simulink library "libraryMatlab"  (R2020b)
settings: Solver=VariableStepAuto  StartTime=0.0  StopTime=10.0  RelTol=1e-3
values from neighbouring files (symbols this model uses):
  data = struct()    [config.m]
undefined symbols (not defined in the file or in its folder): a, SRP
libraries: simulink x2
settings Model: Creator=pacif  LastModifiedBy=pacif

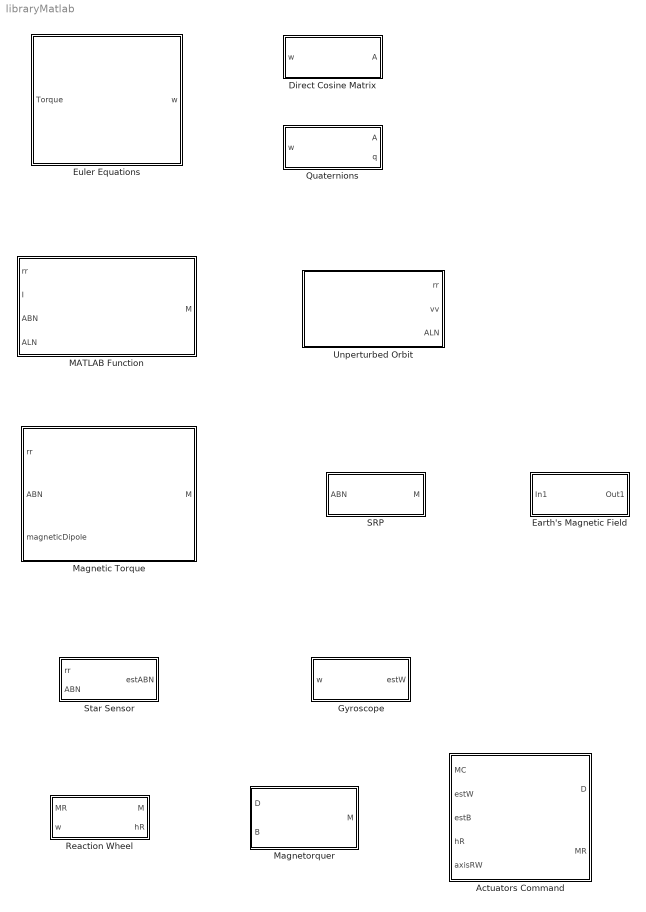
== system libraryMatlab ==
  Actuators Command : MATLAB Function  TreatAsAtomicUnit=on
  Direct Cosine Matrix : Subsystem
  Earth's Magnetic Field : Subsystem
  Euler Equations : Subsystem
  Gyroscope : Subsystem
  MATLAB Function : MATLAB Function  TreatAsAtomicUnit=on
  Magnetic Torque : Subsystem
  Magnetorquer : MATLAB Function  TreatAsAtomicUnit=on
  Quaternions : Subsystem
  Reaction Wheel : Subsystem
  SRP : Subsystem  AncestorBlock=a/SRP
  Star Sensor : Subsystem
  Unperturbed Orbit : Subsystem

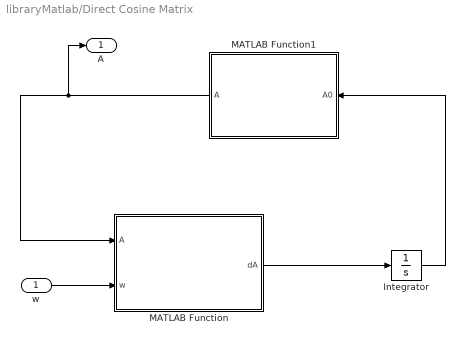
== system libraryMatlab/Direct Cosine Matrix ==
  w : Inport
  Integrator : Integrator  InitialCondition=data.ic.dcm
  MATLAB Function : MATLAB Function  TreatAsAtomicUnit=on
  MATLAB Function1 : MATLAB Function  TreatAsAtomicUnit=on
  A : Outport
  wires:
  w/1 -> MATLAB Function/2(w)
  MATLAB Function/1(dA) -> Integrator/1
  Integrator/1 -> MATLAB Function1/1(A0)
  MATLAB Function1/1(A) -> A/1, MATLAB Function/1(A)

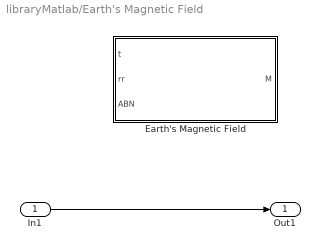
== system libraryMatlab/Earth's Magnetic Field ==
  In1 : Inport
  Earth's Magnetic Field : MATLAB Function  TreatAsAtomicUnit=on
  Out1 : Outport
  wires:
  In1/1 -> Out1/1

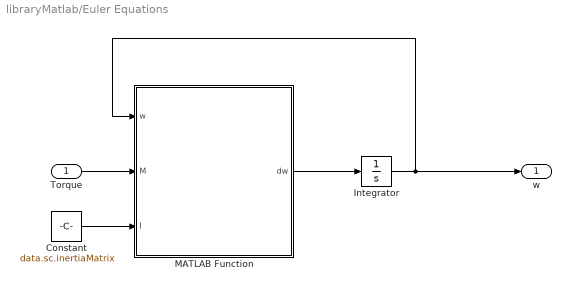
== system libraryMatlab/Euler Equations ==
  Torque : Inport
  Constant : Constant  Value=data.sc.inertiaMatrix
  Integrator : Integrator  InitialCondition=data.ic.w
  MATLAB Function : MATLAB Function  TreatAsAtomicUnit=on
  w : Outport
  wires:
  Constant/1 -> MATLAB Function/3(I)
  Integrator/1 -> w/1, MATLAB Function/1(w)
  Torque/1 -> MATLAB Function/2(M)
  MATLAB Function/1(dw) -> Integrator/1

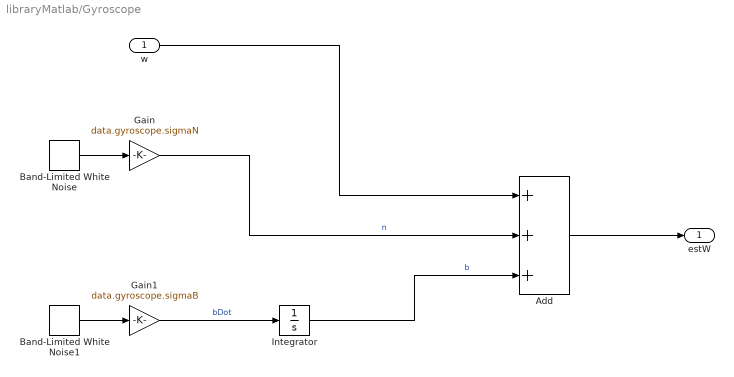
== system libraryMatlab/Gyroscope ==
  w : Inport
  Add : Sum  Inputs=+++
  Band-Limited White Noise : simulink/Sources/Band-Limited White Noise  Cov=[1; 1; 1]  Ts=data.gyroscope.sampleTime  seed=[23341]
  Band-Limited White Noise1 : simulink/Sources/Band-Limited White Noise  Cov=[1; 1; 1]  Ts=data.gyroscope.sampleTime  seed=[23341]
  Gain : Gain  Gain=data.gyroscope.sigmaN
  Gain1 : Gain  Gain=data.gyroscope.sigmaB
  Integrator : Integrator  InitialCondition=[0;0;0]
  estW : Outport
  wires:
  Band-Limited White Noise/1 -> Gain/1
  Gain/1 -> Add/2  "n"
  Gain1/1 -> Integrator/1  "bDot"
  Integrator/1 -> Add/3  "b"
  w/1 -> Add/1
  Add/1 -> estW/1
  Band-Limited White Noise1/1 -> Gain1/1

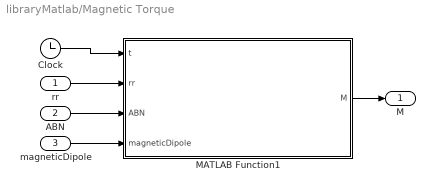
== system libraryMatlab/Magnetic Torque ==
  rr : Inport
  ABN : Inport  Port=2
  magneticDipole : Inport  Port=3
  Clock : Clock
  MATLAB Function1 : MATLAB Function  TreatAsAtomicUnit=on
  M : Outport
  wires:
  MATLAB Function1/1(M) -> M/1
  rr/1 -> MATLAB Function1/2(rr)
  ABN/1 -> MATLAB Function1/3(ABN)
  magneticDipole/1 -> MATLAB Function1/4(magneticDipole)
  Clock/1 -> MATLAB Function1/1(t)

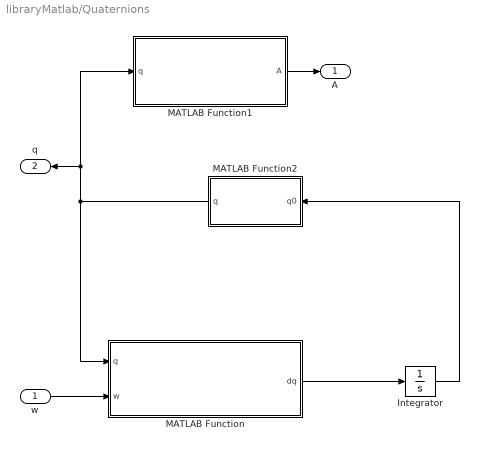
== system libraryMatlab/Quaternions ==
  w : Inport
  Integrator : Integrator  InitialCondition=data.ic.quaternions
  MATLAB Function : MATLAB Function  TreatAsAtomicUnit=on
  MATLAB Function1 : MATLAB Function  TreatAsAtomicUnit=on
  MATLAB Function2 : MATLAB Function  TreatAsAtomicUnit=on
  A : Outport
  q : Outport  Port=2
  wires:
  w/1 -> MATLAB Function/2(w)
  MATLAB Function/1(dq) -> Integrator/1
  Integrator/1 -> MATLAB Function2/1(q0)
  MATLAB Function2/1(q) -> MATLAB Function/1(q), q/1, MATLAB Function1/1(q)
  MATLAB Function1/1(A) -> A/1

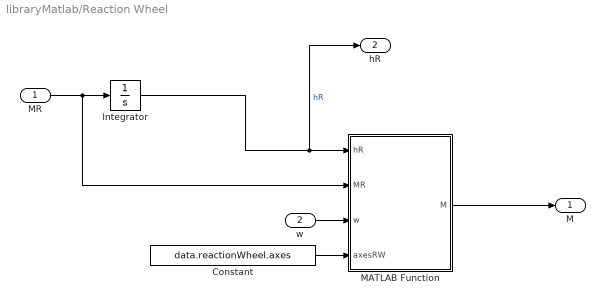
== system libraryMatlab/Reaction Wheel ==
  MR : Inport
  w : Inport  Port=2
  Constant : Constant  Value=data.reactionWheel.axes
  Integrator : Integrator
  MATLAB Function : MATLAB Function  TreatAsAtomicUnit=on
  M : Outport
  hR : Outport  Port=2
  wires:
  MR/1 -> MATLAB Function/2(MR), Integrator/1
  Integrator/1 -> hR/1, MATLAB Function/1(hR)  "hR"
  Constant/1 -> MATLAB Function/4(axesRW)
  w/1 -> MATLAB Function/3(w)
  MATLAB Function/1(M) -> M/1

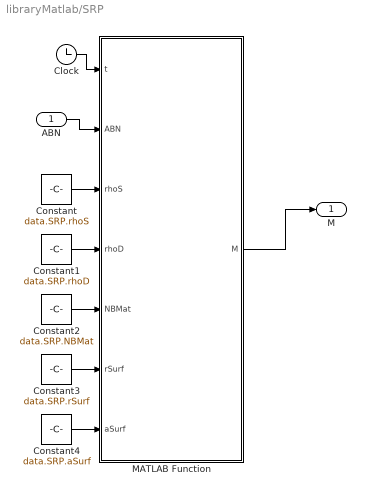
== system libraryMatlab/SRP ==
  ABN : Inport
  Clock : Clock
  Constant : Constant  Value=data.SRP.rhoS
  Constant1 : Constant  Value=data.SRP.rhoD
  Constant2 : Constant  Value=data.SRP.NBMat
  Constant3 : Constant  Value=data.SRP.rSurf
  Constant4 : Constant  Value=data.SRP.aSurf
  MATLAB Function : MATLAB Function  TreatAsAtomicUnit=on
  M : Outport
  wires:
  Constant4/1 -> MATLAB Function/7(aSurf)
  Constant3/1 -> MATLAB Function/6(rSurf)
  Constant2/1 -> MATLAB Function/5(NBMat)
  Constant1/1 -> MATLAB Function/4(rhoD)
  Constant/1 -> MATLAB Function/3(rhoS)
  Clock/1 -> MATLAB Function/1(t)
  MATLAB Function/1(M) -> M/1
  ABN/1 -> MATLAB Function/2(ABN)

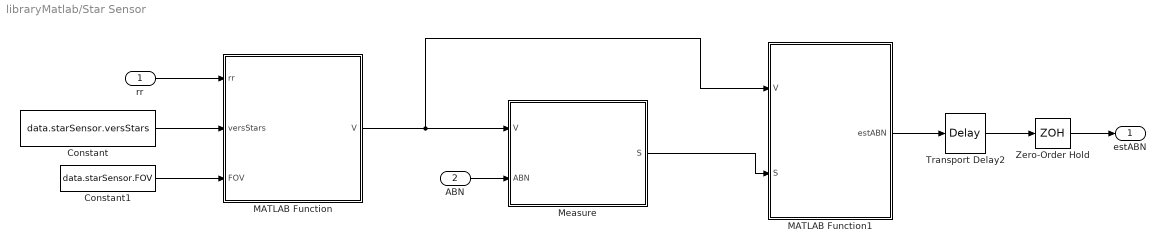
== system libraryMatlab/Star Sensor ==
  rr : Inport
  ABN : Inport  Port=2
  Constant : Constant  Value=data.starSensor.versStars
  Constant1 : Constant  Value=data.starSensor.FOV
  MATLAB Function : MATLAB Function  TreatAsAtomicUnit=on
  MATLAB Function1 : MATLAB Function  TreatAsAtomicUnit=on
  Measure : Subsystem
  Transport Delay2 : TransportDelay  DelayTime=data.starSensor.sampleTime
  Zero-Order Hold : ZeroOrderHold  SampleTime=data.starSensor.sampleTime
  estABN : Outport
  wires:
  Constant/1 -> MATLAB Function/2(versStars)
  Constant1/1 -> MATLAB Function/3(FOV)
  Measure/1(S) -> MATLAB Function1/2(S)
  ABN/1 -> Measure/2(ABN)
  Zero-Order Hold/1 -> estABN/1
  rr/1 -> MATLAB Function/1(rr)
  MATLAB Function/1(V) -> MATLAB Function1/1(V), Measure/1(V)
  MATLAB Function1/1(estABN) -> Transport Delay2/1
  Transport Delay2/1 -> Zero-Order Hold/1

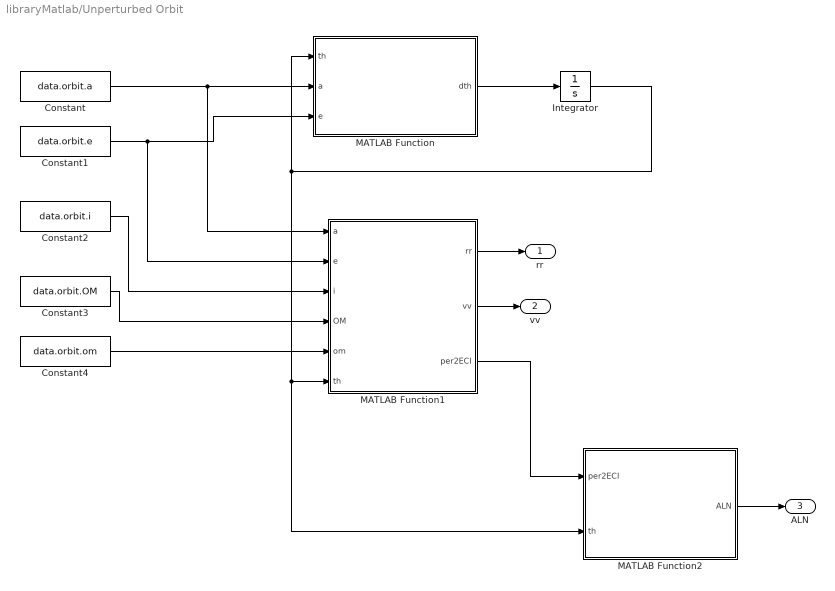
== system libraryMatlab/Unperturbed Orbit ==
  Constant : Constant  Value=data.orbit.a
  Constant1 : Constant  Value=data.orbit.e
  Constant2 : Constant  Value=data.orbit.i
  Constant3 : Constant  Value=data.orbit.OM
  Constant4 : Constant  Value=data.orbit.om
  Integrator : Integrator  InitialCondition=data.ic.th
  MATLAB Function : MATLAB Function  TreatAsAtomicUnit=on
  MATLAB Function1 : MATLAB Function  TreatAsAtomicUnit=on
  MATLAB Function2 : MATLAB Function  TreatAsAtomicUnit=on
  rr : Outport
  vv : Outport  Port=2
  ALN : Outport  Port=3
  wires:
  Constant/1 -> MATLAB Function1/1(a), MATLAB Function/2(a)
  Constant1/1 -> MATLAB Function1/2(e), MATLAB Function/3(e)
  MATLAB Function/1(dth) -> Integrator/1
  Integrator/1 -> MATLAB Function2/2(th), MATLAB Function1/6(th), MATLAB Function/1(th)
  Constant2/1 -> MATLAB Function1/3(i)
  Constant3/1 -> MATLAB Function1/4(OM)
  Constant4/1 -> MATLAB Function1/5(om)
  MATLAB Function1/1(rr) -> rr/1
  MATLAB Function1/2(vv) -> vv/1
  MATLAB Function1/3(per2ECI) -> MATLAB Function2/1(per2ECI)
  MATLAB Function2/1(ALN) -> ALN/1

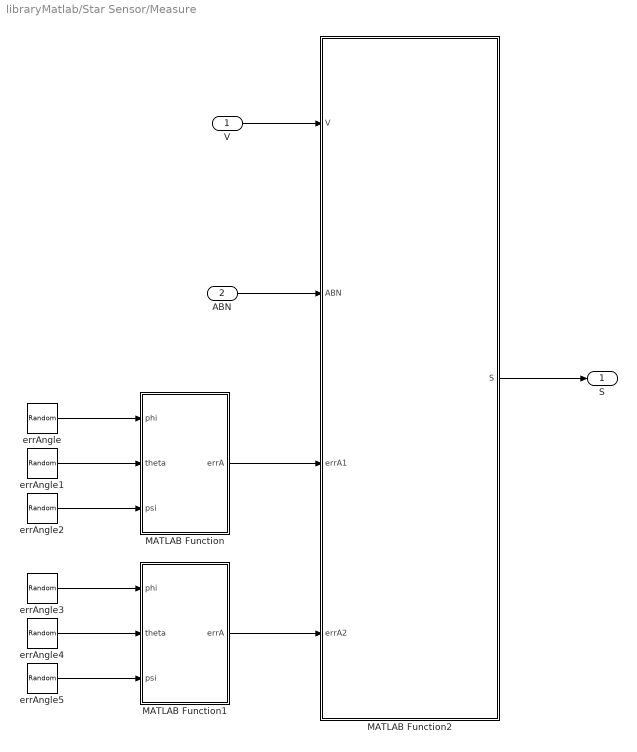
== system libraryMatlab/Star Sensor/Measure ==
  V : Inport
  ABN : Inport  Port=2
  MATLAB Function : MATLAB Function  TreatAsAtomicUnit=on
  MATLAB Function1 : MATLAB Function  TreatAsAtomicUnit=on
  MATLAB Function2 : MATLAB Function  TreatAsAtomicUnit=on
  errAngle{,1..5} (6 alike) : RandomNumber  Variance=data.starSensor.variance  SampleTime=data.starSensor.sampleTime
  S : Outport
  wires:
  errAngle/1 -> MATLAB Function/1(phi)
  errAngle1/1 -> MATLAB Function/2(theta)
  errAngle2/1 -> MATLAB Function/3(psi)
  errAngle5/1 -> MATLAB Function1/3(psi)
  errAngle4/1 -> MATLAB Function1/2(theta)
  errAngle3/1 -> MATLAB Function1/1(phi)
  MATLAB Function/1(errA) -> MATLAB Function2/3(errA1)
  MATLAB Function1/1(errA) -> MATLAB Function2/4(errA2)
  MATLAB Function2/1(S) -> S/1
  V/1 -> MATLAB Function2/1(V)
  ABN/1 -> MATLAB Function2/2(ABN)

== matlab function libraryMatlab/Magnetic Torque/MATLAB Function1 ==
  data: t input; M output; rr input; ABN input; magneticDipole input
function M = magneticTorque(t,rr,ABN,magneticDipole)

% Coefficients for 2020:
g10 = -29615e-9; g11 = -1728e-9; h11 = 5186e-9;
H0 = sqrt(g10^2 + g11^2 + h11^2);

OBL = 11.5*pi/180;
W_EARTH = (2*pi + 2*pi/365.26)/24/3600;
R_EARTH = 6371.0088;

mVers = [sin(OBL)*cos(W_EARTH*t);
        sin(OBL)*sin(W_EARTH*t);
        cos(OBL)];

rVers = rr/norm(rr);
rNorm = norm(rr);

bN = R_EARTH^3/rNorm^3*H0*(3*dot(mVers,rVers)*rVers - mVers);

bB = ABN*bN;

M = cross(magneticDipole,bB); 

end

== matlab function libraryMatlab/SRP/MATLAB Function ==
  data: t input; ABN input; M output; rhoS input; rhoD input; NBMat input; rSurf input; aSurf input
function M = SRP(t,ABN,rhoS,rhoD,NBMat,rSurf,aSurf)

% Constants:
Fe = 2081.4; c = 3e8; P = Fe/c;

N_SUN = 2*pi/365/24/3600; OBL = 23.45*pi/180;
R_SUN = 1.496e8;

SN = R_SUN*[cos(N_SUN*t); 
    sin(N_SUN*t)*cos(OBL);
    sin(N_SUN*t)*sin(OBL)];
SN = SN/norm(SN);

SB = ABN*SN;

nSurf = size(NBMat,2);

M = [0; 0; 0];

for i = 1:nSurf
    
    NBi = NBMat(:,i); ri = rSurf(:,i); Ai = aSurf(i);
    rhoSi = rhoS(i); rhoDi = rhoD(i);
    
    Ki = dot(SB,NBi); 
    
    if Ki > 0
        
        Fi = -P*Ai*Ki*((1-rhoSi)*SB +...
            (2*rhoSi*Ki + 2/3*rhoDi)*NBi);
        
        M = M + cross(ri,Fi);
        
    end
    
end

end

== matlab function libraryMatlab/Star Sensor/MATLAB Function ==
  data: rr input; V output; versStars input; FOV input
function V = starCatalog(rr,versStars,FOV)

rrVers = rr/norm(rr);

% Search on star catalogue:

angles = acos(versStars*rrVers);

anglesInFOV = angles < FOV;

starsInFOV = versStars(anglesInFOV,:);

nMeasures = 2;

V = starsInFOV(1:nMeasures,:)';

== matlab function libraryMatlab/Star Sensor/MATLAB Function1 ==
  data: V input; estABN output; S input
function estABN = attitudeEstimation(V,S)

p = S(:,1); q = S(:,2); a = V(:,1); b = V(:,2);

m1 = p; 
m2 = cross(p,q); m2 = m2/norm(m2);
m3 = cross(p,m2);

n1 = a; 
n2 = cross(a,b); n2 = n2/norm(n2);
n3 = cross(a,n2);

M = [m1, m2, m3]; N = [n1, n2, n3];

estABN = M*N';

== matlab function libraryMatlab/Direct Cosine Matrix/MATLAB Function ==
  data: A input; dA output; w input
function dA = derivativeDCM(A,w)

M = [ 0 -w(3) w(2); 
    w(3) 0 -w(1);
    -w(2) w(1) 0];

dA = -M*A;


end

== matlab function libraryMatlab/Star Sensor/Measure/MATLAB Function ==
  data: phi input; errA output; theta input; psi input
function errA = errorRotation(phi,theta,psi)

errA = [ cos(psi)*cos(theta), cos(phi)*sin(psi) + cos(psi)*sin(phi)*sin(theta), sin(phi)*sin(psi) - cos(phi)*cos(psi)*sin(theta)
-cos(theta)*sin(psi), cos(phi)*cos(psi) - sin(phi)*sin(psi)*sin(theta), cos(psi)*sin(phi) + cos(phi)*sin(psi)*sin(theta)
          sin(theta),                             -cos(theta)*sin(phi),                              cos(phi)*cos(theta)];

== matlab function libraryMatlab/Star Sensor/Measure/MATLAB Function1 ==
  data: phi input; errA output; theta input; psi input
function errA = errorRotation(phi,theta,psi)

errA = [ cos(psi)*cos(theta), cos(phi)*sin(psi) + cos(psi)*sin(phi)*sin(theta), sin(phi)*sin(psi) - cos(phi)*cos(psi)*sin(theta)
-cos(theta)*sin(psi), cos(phi)*cos(psi) - sin(phi)*sin(psi)*sin(theta), cos(psi)*sin(phi) + cos(phi)*sin(psi)*sin(theta)
          sin(theta),                             -cos(theta)*sin(phi),                              cos(phi)*cos(theta)];

== matlab function libraryMatlab/Star Sensor/Measure/MATLAB Function2 ==
  data: V input; S output; ABN input; errA1 input; errA2 input
function S = measure(V,ABN,errA1,errA2)

r1 = V(:,1); r2 = V(:,2);

s1 = errA1*ABN*r1; s2 = errA2*ABN*r2;

S = [s1, s2];

== matlab function libraryMatlab/Reaction Wheel/MATLAB Function ==
  data: hR input; M output; MR input; w input; axesRW input
function M = reactionWheel(hR,MR,w,axesRW)

M = -cross(w,axesRW*hR) - A*MR;

end

== matlab function libraryMatlab/Magnetorquer ==
  data: D input; M output; B input
function M = magnetorquer(D,B)

M = cross(D,B);

end

== matlab function libraryMatlab/Actuators Command ==
  data: MC input; D output; estW input; estB input; hR input; axisRW input; MR output
function [D,MR] = actuatorsCommand(MC, estW, estB, hR, axisRW)

M = MC + cross(estW,hR*axisRW);

Bx = estB(1); By = estB(2); Bz = estB(3);
ax = axisRW(1); ay = axisRW(2); az = axisRW(3);

C = [0, Bz, -By, -ax
     -Bz, 0, Bx, -ay
     By, -Bx, 0, -az];
 
invC = C'*inv(C*C');

u = invC*M;

D = u(1:3); MR = u(4);

end

== matlab function libraryMatlab/Earth's Magnetic Field/Earth's Magnetic Field ==
  data: t input; M output; rr input; ABN input
function M = fcn(t,rr,ABN)

% Coefficients for 2020:
g10 = -29615e-9; g11 = -1728e-9; h11 = 5186e-9;
H0 = sqrt(g10^2 + g11^2 + h11^2);

OBL = 11.5*pi/180;
W_EARTH = (2*pi + 2*pi/365.26)/24/3600;
R_EARTH = 6371.0088;

mVers = [sin(OBL)*cos(W_EARTH*t);
        sin(OBL)*sin(W_EARTH*t);
        cos(OBL)];

rVers = rr/norm(rr);
rNorm = norm(rr);

bN = R_EARTH^3/rNorm^3*H0*(3*dot(mVers,rVers)*rVers - mVers);

bB = ABN*bN;

end

== matlab function libraryMatlab/Euler Equations/MATLAB Function ==
  data: w input; dw output; M input; I input
function dw = eulerEquations(w,M,I)

dw = I\(cross(I*w,w) + M);

end

== matlab function libraryMatlab/Direct Cosine Matrix/MATLAB Function1 ==
  data: A0 input; A output
function A = orthonormalizeA(A0)

A = A0*3/2 - A0*(A0')*A0/2;

end

== matlab function libraryMatlab/Quaternions/MATLAB Function ==
  data: q input; dq output; w input
function dq = derivativeQuaternions(q,w)

w1 = w(1); w2 = w(2); w3 = w(3);

M = [0 w3 -w2 w1; 
    -w3 0 w1 w2;
    w2 -w1 0 w3;
    -w1 -w2 -w3 0];

dq = 0.5*M*q;

end

== matlab function libraryMatlab/Quaternions/MATLAB Function1 ==
  data: q input; A output
function A = quatToDCM(q)

q1 = q(1); q2 = q(2); q3 = q(3); q4 = q(4);

A = [ q1^2-q2^2-q3^2+q4^2    2*(q1*q2+q3*q4)        2*(q1*q3-q2*q4);
    2*(q1*q2-q3*q4)          -q1^2+q2^2-q3^2+q4^2   2*(q2*q3+q1*q4);
    2*(q1*q3+q2*q4)          2*(q2*q3-q1*q4)        -q1^2-q2^2+q3^2+q4^2];

end

== matlab function libraryMatlab/Quaternions/MATLAB Function2 ==
  data: q0 input; q output
function q = normalizeQuat(q0)

q = q0/norm(q0);
q = q0;

end

== matlab function libraryMatlab/MATLAB Function ==
  data: rr input; M output; I input; ABN input; ALN input
function M = gravityGradientTorque(rr,I,ABN,ALN)

MU = 398600;

Ix = I(1,1); Iy = I(2,2); Iz = I(3,3);

R = norm(rr);

ABL = ABN*ALN';

c = ABL*[1;0;0];

K = 3*MU/R^3;

M = K*[ (Iz - Iy)*c(3)*c(2);
        (Ix - Iz)*c(1)*c(3);
        (Iy - Ix)*c(2)*c(1)  ];
    
end

== matlab function libraryMatlab/Unperturbed Orbit/MATLAB Function ==
  data: th input; dth output; a input; e input
function dth = thetaDot(th, a, e)

MU = 398600;

n = sqrt(MU/a^3);

dth = n*(1 + e*cos(th))^2/(1 - e^2)^(3/2);

end

== matlab function libraryMatlab/Unperturbed Orbit/MATLAB Function1 ==
  data: a input; rr output; e input; i input; OM input; om input; th input; vv output; per2ECI output
function [rr,vv,per2ECI] = kep2car(a,e,i,OM,om,th)

MU = 398600;

p = a*(1-e^2);
r = p/(1+e*cos(th));

rr = r*[cos(th);sin(th);0];
vv = sqrt(MU/p)*[-sin(th);e+cos(th);0];

ROM = [ cos(OM) sin(OM) 0; -sin(OM) cos(OM) 0; 0 0 1];
Ri = [ 1 0 0; 0 cos(i) sin(i); 0 -sin(i) cos(i)];
Rom = [ cos(om) sin(om) 0; -sin(om) cos(om) 0; 0 0 1];

per2ECI = (Rom*Ri*ROM)';

rr = per2ECI*rr;
vv = per2ECI*vv;

end

== matlab function libraryMatlab/Unperturbed Orbit/MATLAB Function2 ==
  data: per2ECI input; ALN output; th input
function ALN = computeALN(per2ECI,th)

ECI2per = per2ECI';

per2L = [cos(th)  sin(th)  0;
        -sin(th)  cos(th)  0;
            0        0     1];
        
ALN = per2L*ECI2per;

end
